simulink model "lab3_z"  (R2018b)
settings: Solver=VariableStepAuto  StartTime=0.0  StopTime=t_max  MaxStep=0.1  RelTol=1e-3
undefined symbols (not defined in the file): d, Lo, Lrz, Mo, Mrz, t0, y0
settings Model: Creator=lev  LastModifiedBy=lev

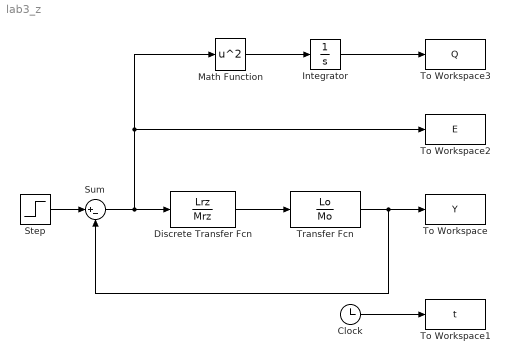
== system lab3_z ==
  Clock : Clock
  Discrete Transfer Fcn : DiscreteTransferFcn  Numerator=Lrz  Denominator=Mrz  SampleTime=d
  Integrator : Integrator
  Math Function : Math  Operator=square  SaturateOnIntegerOverflow=on
  Step : Step  Time=t0  After=y0  SampleTime=0
  Sum : Sum  Inputs=|+-
  To Workspace : ToWorkspace  VariableName=Y  SampleTime=-1
  To Workspace1 : ToWorkspace  VariableName=t  SampleTime=-1
  To Workspace2 : ToWorkspace  VariableName=E  SampleTime=-1
  To Workspace3 : ToWorkspace  VariableName=Q  SampleTime=-1
  Transfer Fcn : TransferFcn  Numerator=Lo  Denominator=Mo
  wires:
  Transfer Fcn/1 -> Sum/2, To Workspace/1
  Clock/1 -> To Workspace1/1
  Sum/1 -> Discrete Transfer Fcn/1, Math Function/1, To Workspace2/1
  Step/1 -> Sum/1
  Math Function/1 -> Integrator/1
  Integrator/1 -> To Workspace3/1
  Discrete Transfer Fcn/1 -> Transfer Fcn/1
